simulink model "PubIfDecisionLM_MDL"  (R2020b)
settings: configuration reference "DspaceConfig" (kept outside this file)
PostLoadFcn:
  | if any(exist('dsrtsu_mdlpostloadfcn', 'file') ~= 0), dsrtsu_mdlpostloadfcn('Execute', bdroot); end
InitFcn:
  | , if any(exist('dsmpb_private', 'file') ~= 0), dsmpb_private('dsmpb_mdlclblib', 'Init', bdroot); end,
undefined symbols (not defined in the file or in its folder): OFM_OBJ_FUSIONTYPE_E, OFM_OBJ_MOVINGSTATE_E, OFM_OBJ_ORIENTATION_E, OFM_OBJ_TYPE_E, P_LM_Cyc, P_LM_EMLHistKapRcdBufSize, P_LM_EMLHistTrajBaseDis, P_LM_EMLHistTrajPNum, P_LM_EMLKapCorrMaxThre, P_LM_EMLMinKapThre, P_LM_EMLPathDisDiffThre, P_LM_EMLQuaFiltPar, P_LM_EMLTurnActKapThre, P_LM_EMLValidQuaThre, P_LM_FntPath1Disgap, P_LM_FntPath1MinDis, P_LM_FntPath1Timegap, P_LM_FntPath2Disgap, P_LM_FntPath2MinDis, P_LM_FntPath2Timegap, P_LM_FntPath3Disgap, P_LM_FntPath3MinDis, P_LM_FntPath3Timegap, P_LM_FusBLParFiltP, P_LM_FusEVDifC2Thre, P_LM_FusEVOPath1AllVSLDisThre, P_LM_FusEVOPath1AllVSLLostNumThre, P_LM_FusEVOPath1AllVSLQuaThre, P_LM_FusEVOPath1OTLFacNLC, P_LM_FusOTLQuaThre, P_LM_FusOTLSW, P_LM_FusParC0Index, P_LM_FusParC1Index, P_LM_FusParC2Index, P_LM_FusParC3Index, P_LM_FusVSLQuaThre, P_LM_FusVSLSW, P_LM_FusVSLValidSteerWheerAngThre, P_LM_FusVSLValidVxvThre, P_LM_LaneWidth, P_LM_OTLBufTPInfoEvaFactor, P_LM_OTLObjNum, P_LM_OTLObjSelectAgeThre, P_LM_OTLObjSelectDxAssessVx, P_LM_OTLObjSelectDxThre, P_LM_OTLObjSelectVxThre, P_LM_OTLObjSelectVyAssessDx, P_LM_OTLObjSelectVyThre, P_LM_OTLTrajPntBaseDis, P_LM_OTLTrajStdThre, P_LM_VSLAvailLineNum, P_LM_VSLBLSDiffThre, P_LM_VSLBLSDisRatio, P_LM_VSLFusBLParFiltP_C1, P_LM_VSLFusBLParFiltP_C2, P_LM_VSLFusBLParFiltP_C3, P_LM_VSLFusBLParFiltP_Quality, P_LM_VSLHistTrajBaseDis, P_LM_VSLHistTrajPNum, P_LM_VSLLCC0diff ... (+18)
libraries: simulink x145, LM_LIB x43
(part 4 of 24)

== system PubIfDecisionLM_MDL/Subsystem2/LM_Fusion1/LM_FusBaseLineInfoCalc/LM_FusBLRearPath ==
  LM_VSL : Inport
  Bus Creator : BusCreator  Inputs=5  OutDataTypeStr=Bus: LM_FusBLPathInfoBus
  Bus Creator1 : BusCreator  Inputs=5  OutDataTypeStr=Bus: LM_FusBLPathInfoBus
  Bus Creator2 : BusCreator  Inputs=5  OutDataTypeStr=Bus: LM_FusBLPathInfoBus
  Bus Selector : BusSelector  OutputSignals=LM_VSLRearPath1P,LM_VSLRearPath1Qulity
  Bus Selector1 : BusSelector  OutputSignals=LM_VSLRearPath2P,LM_VSLRearPath2Qulity
  Bus Selector2 : BusSelector  OutputSignals=LM_VSLRearPath3P,LM_VSLRearPath3Qulity
  LM_EMLRearPath2 : Subsystem
  LM_EMLRearPath3 : Subsystem
  LM_EMLRearPath4 : Subsystem
  Signal Conversion{1..15} (15 alike) : SignalConversion  OverrideOpt=off
  LM_FusBLRearPath1Info : Outport
  LM_FusBLRearPath2Info : Outport  Port=2
  LM_FusBLRearPath3Info : Outport  Port=3
  wires:
  Bus Selector2/2 -> LM_EMLRearPath3/2(LM_VSLRearPath3Quality)  "<LM_VSLRearPath3Qulity>"
  Bus Selector2/1 -> LM_EMLRearPath3/1(LM_VSLRearPath3P)  "<LM_VSLRearPath3P>"
  Bus Selector1/2 -> LM_EMLRearPath2/2(LM_VSLRearPath1Quality)  "<LM_VSLRearPath2Qulity>"
  Bus Selector1/1 -> LM_EMLRearPath2/1(LM_VSLRearPath2P)  "<LM_VSLRearPath2P>"
  Bus Selector/2 -> LM_EMLRearPath4/2(LM_VSLRearPath1Quality)  "<LM_VSLRearPath1Qulity>"
  Bus Selector/1 -> LM_EMLRearPath4/1(LM_VSLRearPath1P)  "<LM_VSLRearPath1P>"
  LM_VSL/1 -> Bus Selector2/1, Bus Selector1/1, Bus Selector/1
  Bus Creator2/1 -> LM_FusBLRearPath3Info/1  "LM_FusBLRearPath3Info"
  Bus Creator1/1 -> LM_FusBLRearPath2Info/1  "LM_FusBLRearPath2Info"
  Bus Creator/1 -> LM_FusBLRearPath1Info/1  "LM_FusBLRearPath1Info"
  LM_EMLRearPath4/3(LM_FusBLRearPath1C2) -> Signal Conversion11/1
  LM_EMLRearPath4/1(LM_FusBLRearPath1C0) -> Signal Conversion9/1
  LM_EMLRearPath4/2(LM_FusBLRearPath1C1) -> Signal Conversion10/1
  Signal Conversion9/1 -> Bus Creator/1  "LM_FusBLPathC0"
  Signal Conversion12/1 -> Bus Creator/4  "LM_FusBLPathC3"
  Signal Conversion10/1 -> Bus Creator/2  "LM_FusBLPathC1"
  Signal Conversion11/1 -> Bus Creator/3  "LM_FusBLPathC2"
  Signal Conversion13/1 -> Bus Creator/5  "LM_FusBLPathQuality"
  LM_EMLRearPath4/4(LM_FusBLRearPath1C3) -> Signal Conversion12/1
  LM_EMLRearPath4/5(LM_FusBLRearPath1Quality) -> Signal Conversion13/1
  LM_EMLRearPath2/5(LM_FusBLRearPath2Quality) -> Signal Conversion4/1
  LM_EMLRearPath2/4(LM_FusBLRearPath2C3) -> Signal Conversion3/1
  Signal Conversion4/1 -> Bus Creator1/5  "LM_FusBLPathQuality"
  Signal Conversion2/1 -> Bus Creator1/3  "LM_FusBLPathC2"
  Signal Conversion1/1 -> Bus Creator1/2  "LM_FusBLPathC1"
  Signal Conversion3/1 -> Bus Creator1/4  "LM_FusBLPathC3"
  Signal Conversion5/1 -> Bus Creator1/1  "LM_FusBLPathC0"
  LM_EMLRearPath2/2(LM_FusBLRearPath2C1) -> Signal Conversion1/1
  LM_EMLRearPath2/1(LM_FusBLRearPath2C0) -> Signal Conversion5/1
  LM_EMLRearPath2/3(LM_FusBLRearPath2C2) -> Signal Conversion2/1
  LM_EMLRearPath3/3(LM_FusBLRearPath3C2) -> Signal Conversion7/1
  LM_EMLRearPath3/1(LM_FusBLRearPath3C0) -> Signal Conversion15/1
  LM_EMLRearPath3/2(LM_FusBLRearPath3C1) -> Signal Conversion6/1
  Signal Conversion15/1 -> Bus Creator2/1  "LM_FusBLPathC0"
  Signal Conversion8/1 -> Bus Creator2/4  "LM_FusBLPathC3"
  Signal Conversion6/1 -> Bus Creator2/2  "LM_FusBLPathC1"
  Signal Conversion7/1 -> Bus Creator2/3  "LM_FusBLPathC2"
  Signal Conversion14/1 -> Bus Creator2/5  "LM_FusBLPathQuality"
  LM_EMLRearPath3/4(LM_FusBLRearPath3C3) -> Signal Conversion8/1
  LM_EMLRearPath3/5(LM_FusBLRearPath3Quality) -> Signal Conversion14/1

== system PubIfDecisionLM_MDL/Subsystem2/LM_Fusion1/LM_FusRatioCalc/LM_FusionCase ==
  note: 0-EML
      | 1-VSL+EML
      | 2-VSL+EML+OTL
      | 3-EML+OTL
  LM_VSLFntPaht1Quality : Inport
  LM_OTLFntPath1Qulity : Inport  Port=2
  LM_OTLFntPath2Qulity : Inport  Port=3
  LM_OTLFntPath3Qulity : Inport  Port=4
  LM_REL : Inport  Port=5
  LM_MAL : Inport  Port=6
  vxvRefMs : Inport  Port=7
  SteerWheelAng : Inport  Port=8
  LM_FusCaseJudge : Subsystem
  LM_FusCaseOTLValidJudge : Subsystem
  LM_FusCaseVSLValidJudge : Subsystem
  Terminator : Terminator
  Terminator1 : Terminator
  LM_FusCase : Outport
  wires:
  LM_REL/1 -> Terminator/1
  LM_MAL/1 -> Terminator1/1
  LM_FusCaseVSLValidJudge/1(LM_FusVSLValid) -> LM_FusCaseJudge/1(LM_FusVSLValid)
  LM_FusCaseOTLValidJudge/1(LM_FusOTLValid) -> LM_FusCaseJudge/2(LM_FusOTLValid)
  LM_FusCaseJudge/1(LM_FusCase) -> LM_FusCase/1
  SteerWheelAng/1 -> LM_FusCaseVSLValidJudge/3(SteerWheelAng)
  LM_VSLFntPaht1Quality/1 -> LM_FusCaseVSLValidJudge/1(LM_VSLFntPaht1Quality)
  vxvRefMs/1 -> LM_FusCaseVSLValidJudge/2(vxvRefMs)
  LM_OTLFntPath3Qulity/1 -> LM_FusCaseOTLValidJudge/3(LM_OTLFntPath3Qulity)
  LM_OTLFntPath2Qulity/1 -> LM_FusCaseOTLValidJudge/2(LM_OTLFntPath2Qulity)
  LM_OTLFntPath1Qulity/1 -> LM_FusCaseOTLValidJudge/1(LM_OTLFntPath1Qulity)

== system PubIfDecisionLM_MDL/Subsystem2/LM_Fusion1/LM_FusRatioCalc/LM_Fusion_EMLOnly ==
  LM_EML : Inport
  Action Port : ActionPort  ActionPortLabel=case [ 0 ]:
  Bus Creator : BusCreator  Inputs=2  OutDataTypeStr=Bus: LM_FusRatioInfoBus  NonVirtualBus=on
  Bus Creator1 : BusCreator  Inputs=4  OutDataTypeStr=Bus: LM_FusC0InfoBus  NonVirtualBus=on
  Bus Selector : BusSelector  OutputSignals=LM_EMLLLC0,LM_EMLLRC0,LM_EMLRLC0,LM_EMLRRC0
  LM_FusBaseLineC0Info : Subsystem
  LM_FusEMLAndVSLRatioCalc : Subsystem
  LM_FusBLInfo : Outport
  LM_C0Info : Outport  Port=2
  wires:
  Bus Selector/2 -> LM_FusBaseLineC0Info/2(LM_EMLC0)  "<LM_EMLLRC0>"
  Bus Selector/4 -> LM_FusBaseLineC0Info/4(LM_EMLRRC0)  "<LM_EMLRRC0>"
  Bus Selector/3 -> LM_FusBaseLineC0Info/3(LM_EMLRLC0)  "<LM_EMLRLC0>"
  LM_EML/1 -> Bus Selector/1
  Bus Creator/1 -> LM_FusBLInfo/1
  Bus Selector/1 -> LM_FusBaseLineC0Info/1(LM_EMLLLC0)  "<LM_EMLLLC0>"
  LM_FusBaseLineC0Info/1(LM_LLC0) -> Bus Creator1/1
  LM_FusBaseLineC0Info/2(LM_LRC0) -> Bus Creator1/2
  LM_FusBaseLineC0Info/3(LM_RLC0) -> Bus Creator1/3
  LM_FusBaseLineC0Info/4(LM_RRC0) -> Bus Creator1/4
  LM_FusEMLAndVSLRatioCalc/1(LM_FusFntPathK) -> Bus Creator/1
  LM_FusEMLAndVSLRatioCalc/2(LM_FusRearPathK) -> Bus Creator/2
  Bus Creator1/1 -> LM_C0Info/1  "LM_C0Info"

== system PubIfDecisionLM_MDL/Subsystem2/LM_Fusion1/LM_FusRatioCalc/LM_Fusion_EO ==
  DIR_BUS : Inport
  LM_EML : Inport  Port=2
  LM_OTL : Inport  Port=3
  LM_Com : Inport  Port=4
  LM_VIE_BUS : Inport  Port=5
  Action Port : ActionPort  ActionPortLabel=case [ 3 ]:
  Bus Creator : BusCreator  Inputs=2  OutDataTypeStr=Bus: LM_FusRatioInfoBus  NonVirtualBus=on
  Bus Creator1 : BusCreator  Inputs=4  OutDataTypeStr=Bus: LM_FusC0InfoBus  NonVirtualBus=on
  Bus Selector : BusSelector  OutputSignals=LM_EMLLLC0,LM_EMLLRC0,LM_EMLRLC0,LM_EMLRRC0
  LM_FusBaseLineC0Info : Subsystem
  LM_FusEVORatioCalc : Subsystem
  LM_FusRatioInfo : Outport
  LM_C0Info : Outport  Port=2
  wires:
  LM_VIE_BUS/1 -> LM_FusEVORatioCalc/5(LM_VIE_BUS)
  LM_OTL/1 -> LM_FusEVORatioCalc/3(LM_OTL)
  Bus Creator/1 -> LM_FusRatioInfo/1  "LM_FusRatioInfo"
  Bus Selector/4 -> LM_FusBaseLineC0Info/4(LM_VSLRRC0Adju)  "<LM_EMLRRC0>"
  LM_Com/1 -> LM_FusEVORatioCalc/4(LM_Com)
  LM_EML/1 -> Bus Selector/1, LM_FusEVORatioCalc/2(LM_EML)
  Bus Selector/2 -> LM_FusBaseLineC0Info/2(LM_VSLLRC0Adju)  "<LM_EMLLRC0>"
  Bus Selector/1 -> LM_FusBaseLineC0Info/1(LM_VSLLLC0Adju)  "<LM_EMLLLC0>"
  Bus Selector/3 -> LM_FusBaseLineC0Info/3(LM_VSLRLC0Adju)  "<LM_EMLRLC0>"
  LM_FusBaseLineC0Info/3(LM_RLC0) -> Bus Creator1/3
  Bus Creator1/1 -> LM_C0Info/1  "LM_C0Info"
  LM_FusBaseLineC0Info/4(LM_RRC0) -> Bus Creator1/4
  LM_FusBaseLineC0Info/1(LM_LLC0) -> Bus Creator1/1
  LM_FusBaseLineC0Info/2(LM_LRC0) -> Bus Creator1/2
  LM_FusEVORatioCalc/1(LM_FusFntPathK) -> Bus Creator/1
  LM_FusEVORatioCalc/2(LM_FusRearPathK) -> Bus Creator/2
  DIR_BUS/1 -> LM_FusEVORatioCalc/1(DIR_BUS)

== system PubIfDecisionLM_MDL/Subsystem2/LM_Fusion1/LM_FusRatioCalc/LM_Fusion_EV ==
  LM_VSL : Inport
  LM_EML : Inport  Port=2
  LM_VIE_BUS : Inport  Port=3
  LM_ComBus : Inport  Port=4
  DIR_BUS : Inport  Port=5
  Action Port : ActionPort  ActionPortLabel=case [ 1 ]:
  Bus Creator : BusCreator  Inputs=2  OutDataTypeStr=Bus: LM_FusRatioInfoBus  NonVirtualBus=on
  Bus Creator1 : BusCreator  Inputs=4  OutDataTypeStr=Bus: LM_FusC0InfoBus  NonVirtualBus=on
  LM_FusBaseLineC0Info : Subsystem
  LM_FusEMLAndVSLRatioCalc : Subsystem
  LM_FusBLInfo : Outport
  LM_C0Info : Outport  Port=2
  wires:
  LM_VSL/1 -> LM_FusBaseLineC0Info/2(LM_VSL), LM_FusEMLAndVSLRatioCalc/4(LM_VSL)
  LM_EML/1 -> LM_FusBaseLineC0Info/3(LM_EML), LM_FusEMLAndVSLRatioCalc/5(LM_EML)
  LM_ComBus/1 -> LM_FusEMLAndVSLRatioCalc/2(LM_ComBus)
  Bus Creator/1 -> LM_FusBLInfo/1  "LM_FusBLInfo"
  LM_FusBaseLineC0Info/4(LM_RRC0) -> Bus Creator1/4
  LM_FusBaseLineC0Info/2(LM_LRC0) -> Bus Creator1/2
  LM_FusBaseLineC0Info/3(LM_RLC0) -> Bus Creator1/3
  LM_FusBaseLineC0Info/1(LM_LLC0) -> Bus Creator1/1
  Bus Creator1/1 -> LM_C0Info/1  "LM_C0Info"
  DIR_BUS/1 -> LM_FusEMLAndVSLRatioCalc/3(DIR_BUS)
  LM_FusEMLAndVSLRatioCalc/2(LM_FusRearPathK) -> Bus Creator/2
  LM_FusEMLAndVSLRatioCalc/1(LM_FusFntPathK) -> LM_FusBaseLineC0Info/1(LM_FusFntPathK), Bus Creator/1
  LM_VIE_BUS/1 -> LM_FusEMLAndVSLRatioCalc/1(LM_VIE_BUS)

== system PubIfDecisionLM_MDL/Subsystem2/LM_Fusion1/LM_FusRatioCalc/LM_Fusion_EVO ==
  LM_VSL : Inport
  LM_EML : Inport  Port=2
  LM_OTL : Inport  Port=3
  LM_Com : Inport  Port=4
  LM_VIE_BUS : Inport  Port=5
  DIR_BUS : Inport  Port=6
  Action Port : ActionPort  ActionPortLabel=case [ 2 ]:
  Bus Creator : BusCreator  Inputs=2  OutDataTypeStr=Bus: LM_FusRatioInfoBus  NonVirtualBus=on
  Bus Creator1 : BusCreator  Inputs=4  OutDataTypeStr=Bus: LM_FusC0InfoBus  NonVirtualBus=on
  Bus Selector : BusSelector  OutputSignals=LM_VSLLLC0,LM_VSLLRC0,LM_VSLRLC0,LM_VSLRRC0
  LM_FusBaseLineC0Info : Subsystem
  LM_FusEVORatioCalc : Subsystem
  LM_FusBLInfo : Outport
  LM_C0Info : Outport  Port=2
  wires:
  Bus Selector/3 -> LM_FusBaseLineC0Info/3(LM_VSLRLC0Adju)  "<LM_VSLRLC0>"
  Bus Selector/1 -> LM_FusBaseLineC0Info/1(LM_VSLLLC0Adju)  "<LM_VSLLLC0>"
  Bus Selector/2 -> LM_FusBaseLineC0Info/2(LM_VSLLRC0Adju)  "<LM_VSLLRC0>"
  LM_EML/1 -> LM_FusEVORatioCalc/2(LM_EML)
  LM_VSL/1 -> Bus Selector/1, LM_FusEVORatioCalc/1(LM_VSL)
  LM_Com/1 -> LM_FusEVORatioCalc/4(LM_Com)
  Bus Selector/4 -> LM_FusBaseLineC0Info/4(LM_VSLRRC0Adju)  "<LM_VSLRRC0>"
  Bus Creator/1 -> LM_FusBLInfo/1  "LM_FusBLInfo"
  LM_OTL/1 -> LM_FusEVORatioCalc/3(LM_OTL)
  LM_VIE_BUS/1 -> LM_FusEVORatioCalc/5(LM_VIE_BUS)
  LM_FusEVORatioCalc/1(LM_FusFntPathK) -> Bus Creator/1
  LM_FusEVORatioCalc/2(LM_FusRearPathK) -> Bus Creator/2
  LM_FusBaseLineC0Info/3(LM_RLC0) -> Bus Creator1/3
  Bus Creator1/1 -> LM_C0Info/1  "LM_C0Info"
  LM_FusBaseLineC0Info/4(LM_RRC0) -> Bus Creator1/4
  LM_FusBaseLineC0Info/1(LM_LLC0) -> Bus Creator1/1
  LM_FusBaseLineC0Info/2(LM_LRC0) -> Bus Creator1/2
  DIR_BUS/1 -> LM_FusEVORatioCalc/6(DIR_BUS)

== system PubIfDecisionLM_MDL/Subsystem2/LM_Fusion1/LM_Fus_BLConnectivityCheck/LM_Fus_BLFntPahtConnectivityCheck ==
  LM_ComBus : Inport
  LM_FusBLInfoFilt : Inport  Port=2
  Bus Creator : BusCreator  Inputs=5  OutDataTypeStr=Bus: LM_FusBLPathInfoBus
  Bus Creator1 : BusCreator  Inputs=5  OutDataTypeStr=Bus: LM_FusBLPathInfoBus
  Bus Creator2 : BusCreator  Inputs=5  OutDataTypeStr=Bus: LM_FusBLPathInfoBus
  Bus Selector : BusSelector  OutputSignals=LM_FusBLFntPath1Info.LM_FusBLPathC0,LM_FusBLFntPath1Info.LM_FusBLPathC1,LM_FusBLFntPath1Info.LM_FusBLPathC2,LM_FusBLFntPath1Info.LM_FusBLPathC3,LM_FusBLFntPath1Info.LM_FusBLPathQuality,LM_FusBLFntPath2Info.LM_FusBLPathC0,LM_FusBLFntPath2Info.LM_FusBLPathC1,LM_FusBLFntPath2Info.LM_FusBLPathC2,LM_FusBLFntPath2Info.LM_FusBLPathC3,LM_FusBLFntPath2Info.LM_FusBLPathQuality,LM_FusBLFntPath3Info.LM_FusBLPathC0,LM_FusBLFntPath3Info.LM_FusBLPathC1,LM_FusBLFntPath3Info.LM_FusBLPathC2,LM_FusBLFntPath3Info.LM_FusBLPathC3,LM_FusBLFntPath3Info.LM_FusBLPathQuality
  Bus Selector1 : BusSelector  OutputSignals=LM_PathDisBus.LM_FntPath1Dis,LM_PathDisBus.LM_FntPath2Dis
  LM_Fus_BLFntPahtConnectivityCheck : Subsystem
  Signal Conversion{,1..14} (15 alike) : SignalConversion  OverrideOpt=off
  LM_FusBLFntPath1Info : Outport
  LM_FusBLFntPath2Info : Outport  Port=2
  LM_FusBLFntPath3Info : Outport  Port=3
  wires:
  LM_FusBLInfoFilt/1 -> Bus Selector/1
  Bus Selector/1 -> LM_Fus_BLFntPahtConnectivityCheck/1(LM_FusBLFntPath1C0)  "<LM_FusBLPathC0>"
  Bus Selector/2 -> LM_Fus_BLFntPahtConnectivityCheck/2(LM_FusBLFntPath1C1)  "<LM_FusBLPathC1>"
  Bus Selector/3 -> LM_Fus_BLFntPahtConnectivityCheck/3(LM_FusBLFntPath1C2)  "<LM_FusBLPathC2>"
  Bus Selector/4 -> LM_Fus_BLFntPahtConnectivityCheck/4(LM_FusBLFntPath1C3)  "<LM_FusBLPathC3>"
  Bus Selector/5 -> LM_Fus_BLFntPahtConnectivityCheck/5(LM_FusBLFntPath1Quality)  "<LM_FusBLPathQuality>"
  Bus Selector/6 -> LM_Fus_BLFntPahtConnectivityCheck/6(LM_FusBLFntPath2C0BefAduj)  "<LM_FusBLPathC0>"
  Bus Selector/7 -> LM_Fus_BLFntPahtConnectivityCheck/7(LM_FusBLFntPath2C1)  "<LM_FusBLPathC1>"
  Bus Selector/8 -> LM_Fus_BLFntPahtConnectivityCheck/8(LM_FusBLFntPath2C2)  "<LM_FusBLPathC2>"
  Bus Selector/9 -> LM_Fus_BLFntPahtConnectivityCheck/9(LM_FusBLFntPath2C3)  "<LM_FusBLPathC3>"
  Bus Selector/10 -> LM_Fus_BLFntPahtConnectivityCheck/10(LM_FusBLFntPath2Quality)  "<LM_FusBLPathQuality>"
  Bus Selector/11 -> LM_Fus_BLFntPahtConnectivityCheck/11(LM_FusBLFntPath3C0BefAduj)  "<LM_FusBLPathC0>"
  Bus Selector/12 -> LM_Fus_BLFntPahtConnectivityCheck/12(LM_FusBLFntPath3C1)  "<LM_FusBLPathC1>"
  Bus Selector/13 -> LM_Fus_BLFntPahtConnectivityCheck/13(LM_FusBLFntPath3C2)  "<LM_FusBLPathC2>"
  Bus Selector/14 -> LM_Fus_BLFntPahtConnectivityCheck/14(LM_FusBLFntPath3C3)  "<LM_FusBLPathC3>"
  Bus Selector/15 -> LM_Fus_BLFntPahtConnectivityCheck/15(LM_FusBLFntPath3Quality)  "<LM_FusBLPathQuality>"
  LM_ComBus/1 -> Bus Selector1/1
  Bus Selector1/1 -> LM_Fus_BLFntPahtConnectivityCheck/16(LM_FntPath1Dis)  "<LM_FntPath1Dis>"
  Bus Selector1/2 -> LM_Fus_BLFntPahtConnectivityCheck/17(LM_FntPath2Dis)  "<LM_FntPath2Dis>"
  LM_Fus_BLFntPahtConnectivityCheck/1(LM_FusBLFntPath1C0Adju) -> Signal Conversion/1
  LM_Fus_BLFntPahtConnectivityCheck/2(LM_FusBLFntPath1C1Adju) -> Signal Conversion1/1
  LM_Fus_BLFntPahtConnectivityCheck/4(LM_FusBLFntPath1C3Adju) -> Signal Conversion3/1
  LM_Fus_BLFntPahtConnectivityCheck/3(LM_FusBLFntPath1C2Adju) -> Signal Conversion2/1
  LM_Fus_BLFntPahtConnectivityCheck/7(LM_FusBLFntPath2C1Adju) -> Signal Conversion6/1
  LM_Fus_BLFntPahtConnectivityCheck/8(LM_FusBLFntPath2C2Adju) -> Signal Conversion7/1
  LM_Fus_BLFntPahtConnectivityCheck/6(LM_FusBLFntPath2C0Adju) -> Signal Conversion5/1
  LM_Fus_BLFntPahtConnectivityCheck/5(LM_FusBLFntPath1QualityAdju) -> Signal Conversion4/1
  LM_Fus_BLFntPahtConnectivityCheck/13(LM_FusBLFntPath3C2Adju) -> Signal Conversion12/1
  LM_Fus_BLFntPahtConnectivityCheck/14(LM_FusBLFntPath3C3Adju) -> Signal Conversion13/1
  LM_Fus_BLFntPahtConnectivityCheck/15(LM_FusBLFntPath3QualityAdju) -> Signal Conversion14/1
  LM_Fus_BLFntPahtConnectivityCheck/11(LM_FusBLFntPath3C0Adju) -> Signal Conversion10/1
  LM_Fus_BLFntPahtConnectivityCheck/12(LM_FusBLFntPath3C1Adju) -> Signal Conversion11/1
  LM_Fus_BLFntPahtConnectivityCheck/10(LM_FusBLFntPath2QualityAdju) -> Signal Conversion9/1
  LM_Fus_BLFntPahtConnectivityCheck/9(LM_FusBLFntPath2C3Adju) -> Signal Conversion8/1
  Bus Creator/1 -> LM_FusBLFntPath1Info/1  "LM_FusBLFntPath1Info"
  Bus Creator1/1 -> LM_FusBLFntPath2Info/1  "LM_FusBLFntPath2Info"
  Bus Creator2/1 -> LM_FusBLFntPath3Info/1  "LM_FusBLFntPath3Info"
  Signal Conversion4/1 -> Bus Creator/5  "LM_FusBLPathQuality"
  Signal Conversion3/1 -> Bus Creator/4  "LM_FusBLPathC3"
  Signal Conversion2/1 -> Bus Creator/3  "LM_FusBLPathC2"
  Signal Conversion1/1 -> Bus Creator/2  "LM_FusBLPathC1"
  Signal Conversion/1 -> Bus Creator/1  "LM_FusBLPathC0"
  Signal Conversion5/1 -> Bus Creator1/1  "LM_FusBLPathC0"
  Signal Conversion6/1 -> Bus Creator1/2  "LM_FusBLPathC1"
  Signal Conversion7/1 -> Bus Creator1/3  "LM_FusBLPathC2"
  Signal Conversion8/1 -> Bus Creator1/4  "LM_FusBLPathC3"
  Signal Conversion9/1 -> Bus Creator1/5  "LM_FusBLPathQuality"
  Signal Conversion14/1 -> Bus Creator2/5  "LM_FusBLPathQuality"
  Signal Conversion13/1 -> Bus Creator2/4  "LM_FusBLPathC3"
  Signal Conversion12/1 -> Bus Creator2/3  "LM_FusBLPathC2"
  Signal Conversion11/1 -> Bus Creator2/2  "LM_FusBLPathC1"
  Signal Conversion10/1 -> Bus Creator2/1  "LM_FusBLPathC0"

== system PubIfDecisionLM_MDL/Subsystem2/LM_Fusion1/LM_Fus_BLConnectivityCheck/LM_Fus_BLRearPahtConnectivityCheck ==
  LM_ComBus : Inport
  LM_FusBLInfoFilt : Inport  Port=2
  Bus Creator : BusCreator  Inputs=5  OutDataTypeStr=Bus: LM_FusBLPathInfoBus
  Bus Creator1 : BusCreator  Inputs=5  OutDataTypeStr=Bus: LM_FusBLPathInfoBus
  Bus Creator3 : BusCreator  Inputs=5  OutDataTypeStr=Bus: LM_FusBLPathInfoBus
  Bus Selector : BusSelector  OutputSignals=LM_FusBLRearPath1Info.LM_FusBLPathC0,LM_FusBLRearPath1Info.LM_FusBLPathC1,LM_FusBLRearPath1Info.LM_FusBLPathC2,LM_FusBLRearPath1Info.LM_FusBLPathC3,LM_FusBLRearPath1Info.LM_FusBLPathQuality,LM_FusBLRearPath2Info.LM_FusBLPathC0,LM_FusBLRearPath2Info.LM_FusBLPathC1,LM_FusBLRearPath2Info.LM_FusBLPathC2,LM_FusBLRearPath2Info.LM_FusBLPathC3,LM_FusBLRearPath2Info.LM_FusBLPathQuality,LM_FusBLRearPath3Info.LM_FusBLPathC0,LM_FusBLRearPath3Info.LM_FusBLPathC1,LM_FusBLRearPath3Info.LM_FusBLPathC2,LM_FusBLRearPath3Info.LM_FusBLPathC3,LM_FusBLRearPath3Info.LM_FusBLPathQuality
  Bus Selector1 : BusSelector  OutputSignals=LM_PathDisBus.LM_RearPath1Dis,LM_PathDisBus.LM_RearPath2Dis
  LM_Fus_BLRearPahtConnectivityCheck : Subsystem
  Signal Conversion{,1..11,14..16} (15 alike) : SignalConversion  OverrideOpt=off
  LM_FusBLFntPath1Info : Outport
  LM_FusBLFntPath2Info : Outport  Port=2
  LM_FusBLFntPath3Info : Outport  Port=3
  wires:
  LM_FusBLInfoFilt/1 -> Bus Selector/1
  Bus Selector/1 -> LM_Fus_BLRearPahtConnectivityCheck/1(LM_FusBLRearPath1C0)  "<LM_FusBLPathC0>"
  Bus Selector/2 -> LM_Fus_BLRearPahtConnectivityCheck/2(LM_FusBLRearPath1C1)  "<LM_FusBLPathC1>"
  Bus Selector/3 -> LM_Fus_BLRearPahtConnectivityCheck/3(LM_FusBLRearPath1C2)  "<LM_FusBLPathC2>"
  Bus Selector/4 -> LM_Fus_BLRearPahtConnectivityCheck/4(LM_FusBLRearPath1C3)  "<LM_FusBLPathC3>"
  Bus Selector/5 -> LM_Fus_BLRearPahtConnectivityCheck/5(LM_FusBLRearPath1Quality)  "<LM_FusBLPathQuality>"
  Bus Selector/6 -> LM_Fus_BLRearPahtConnectivityCheck/6(LM_FusBLRearPath2C0BefAduj)  "<LM_FusBLPathC0>"
  Bus Selector/7 -> LM_Fus_BLRearPahtConnectivityCheck/7(LM_FusBLRearPath2C1)  "<LM_FusBLPathC1>"
  Bus Selector/8 -> LM_Fus_BLRearPahtConnectivityCheck/8(LM_FusBLRearPath2C2)  "<LM_FusBLPathC2>"
  Bus Selector/9 -> LM_Fus_BLRearPahtConnectivityCheck/9(LM_FusBLRearPath2C3)  "<LM_FusBLPathC3>"
  Bus Selector/10 -> LM_Fus_BLRearPahtConnectivityCheck/10(LM_FusBLRearPath2Quality)  "<LM_FusBLPathQuality>"
  Bus Selector/11 -> LM_Fus_BLRearPahtConnectivityCheck/11(LM_FusBLRearPath3C0BefAduj)  "<LM_FusBLPathC0>"
  Bus Selector/12 -> LM_Fus_BLRearPahtConnectivityCheck/12(LM_FusBRearPath3C1)  "<LM_FusBLPathC1>"
  Bus Selector/13 -> LM_Fus_BLRearPahtConnectivityCheck/13(LM_FusBLRearPath3C2)  "<LM_FusBLPathC2>"
  Bus Selector/14 -> LM_Fus_BLRearPahtConnectivityCheck/14(LM_FusBLRearPath3C3)  "<LM_FusBLPathC3>"
  Bus Selector/15 -> LM_Fus_BLRearPahtConnectivityCheck/15(LM_FusBLRearPath3Quality)  "<LM_FusBLPathQuality>"
  LM_ComBus/1 -> Bus Selector1/1
  Bus Selector1/1 -> LM_Fus_BLRearPahtConnectivityCheck/16(LM_RearPath1Dis)  "<LM_RearPath1Dis>"
  Bus Selector1/2 -> LM_Fus_BLRearPahtConnectivityCheck/17(LM_RearPath2Dis)  "<LM_RearPath2Dis>"
  LM_Fus_BLRearPahtConnectivityCheck/1(LM_FusBLRearPath1C0Adju) -> Signal Conversion/1
  LM_Fus_BLRearPahtConnectivityCheck/2(LM_FusBLRearPath1C1Adju) -> Signal Conversion1/1
  LM_Fus_BLRearPahtConnectivityCheck/3(LM_FusBLRearPath1C2Adju) -> Signal Conversion2/1
  LM_Fus_BLRearPahtConnectivityCheck/6(LM_FusBLRearPath2C0Adju) -> Signal Conversion5/1
  LM_Fus_BLRearPahtConnectivityCheck/5(LM_FusBLRearPath1QualityAdju) -> Signal Conversion4/1
  LM_Fus_BLRearPahtConnectivityCheck/4(LM_FusBLRearPath1C3Adju) -> Signal Conversion3/1
  LM_Fus_BLRearPahtConnectivityCheck/10(LM_FusBLRearPath2QualityAdju) -> Signal Conversion9/1
  LM_Fus_BLRearPahtConnectivityCheck/11(LM_FusBLRearPath3C0Adju) -> Signal Conversion10/1
  LM_Fus_BLRearPahtConnectivityCheck/12(LM_FusBLRearPath3C1Adju) -> Signal Conversion11/1
  LM_Fus_BLRearPahtConnectivityCheck/9(LM_FusBLRearPath2C3Adju) -> Signal Conversion8/1
  LM_Fus_BLRearPahtConnectivityCheck/8(LM_FusBLRearPath2C2Adju) -> Signal Conversion7/1
  LM_Fus_BLRearPahtConnectivityCheck/7(LM_FusBLRearPath2C1Adju) -> Signal Conversion6/1
  LM_Fus_BLRearPahtConnectivityCheck/13(LM_FusBLRearPath3C2Adju) -> Signal Conversion14/1
  LM_Fus_BLRearPahtConnectivityCheck/14(LM_FusBLRearPath3C3Adju) -> Signal Conversion15/1
  LM_Fus_BLRearPahtConnectivityCheck/15(LM_FusBLRearPath3QualityAdju) -> Signal Conversion16/1
  Bus Creator3/1 -> LM_FusBLFntPath3Info/1  "LM_FusBLRearPath3Info"
  Bus Creator1/1 -> LM_FusBLFntPath2Info/1  "LM_FusBLRearPath2Info"
  Bus Creator/1 -> LM_FusBLFntPath1Info/1  "LM_FusBLRearPath1Info"
  Signal Conversion4/1 -> Bus Creator/5  "LM_FusBLPathQuality"
  Signal Conversion3/1 -> Bus Creator/4  "LM_FusBLPathC3"
  Signal Conversion2/1 -> Bus Creator/3  "LM_FusBLPathC2"
  Signal Conversion1/1 -> Bus Creator/2  "LM_FusBLPathC1"
  Signal Conversion/1 -> Bus Creator/1  "LM_FusBLPathC0"
  Signal Conversion5/1 -> Bus Creator1/1  "LM_FusBLPathC0"
  Signal Conversion6/1 -> Bus Creator1/2  "LM_FusBLPathC1"
  Signal Conversion7/1 -> Bus Creator1/3  "LM_FusBLPathC2"
  Signal Conversion8/1 -> Bus Creator1/4  "LM_FusBLPathC3"
  Signal Conversion9/1 -> Bus Creator1/5  "LM_FusBLPathQuality"
  Signal Conversion16/1 -> Bus Creator3/5  "LM_FusBLPathQuality"
  Signal Conversion15/1 -> Bus Creator3/4  "LM_FusBLPathC3"
  Signal Conversion14/1 -> Bus Creator3/3  "LM_FusBLPathC2"
  Signal Conversion11/1 -> Bus Creator3/2  "LM_FusBLPathC1"
  Signal Conversion10/1 -> Bus Creator3/1  "LM_FusBLPathC0"

== system PubIfDecisionLM_MDL/Subsystem2/LM_Fusion1/LM_FusfCamValidInfoCalc/LM_FusfCamValidInfoCalc ==
  LM_FusFntPath1VSLK : Inport
  LM_FusFntPath2VSLK : Inport  Port=2
  LM_FusFntPath3VSLK : Inport  Port=3
  Compare To Zero : simulink/Logic and Bit Operations/Compare To Zero  relop=~=  OutDataTypeStr=boolean
  Compare To Zero1 : simulink/Logic and Bit Operations/Compare To Zero  relop=~=  OutDataTypeStr=boolean
  Compare To Zero2 : simulink/Logic and Bit Operations/Compare To Zero  relop=~=  OutDataTypeStr=boolean
  Constant : Constant  OutDataTypeStr=uint8
  Constant1 : Constant  Value=0  OutDataTypeStr=uint8
  Switch : Switch  Criteria=u2 ~= 0
  Switch1 : Switch  Criteria=u2 ~= 0
  Switch2 : Switch  Criteria=u2 ~= 0
  LM_FusFntPath1fCamValid : Outport
  LM_FusFntPath2fCamValid : Outport  Port=2
  LM_FusFntPath3fCamValid : Outport  Port=3
  wires:
  Compare To Zero/1 -> Switch/2
  LM_FusFntPath1VSLK/1 -> Compare To Zero/1
  Compare To Zero1/1 -> Switch1/2
  Compare To Zero2/1 -> Switch2/2
  LM_FusFntPath3VSLK/1 -> Compare To Zero2/1
  LM_FusFntPath2VSLK/1 -> Compare To Zero1/1
  Constant/1 -> Switch2/1, Switch1/1, Switch/1
  Constant1/1 -> Switch/3, Switch2/3, Switch1/3
  Switch/1 -> LM_FusFntPath1fCamValid/1  "LM_FusFntPath1fCamValid"
  Switch1/1 -> LM_FusFntPath2fCamValid/1  "LM_FusFntPath2fCamValid"
  Switch2/1 -> LM_FusFntPath3fCamValid/1  "LM_FusFntPath3fCamValid"

== system PubIfDecisionLM_MDL/Subsystem2/LM_OTL/LM_OTL_MovObjTrajFit/LM_OTL_BufTPAssess ==
  LM_OTLBufTPInfoBus : Inport
  LM_OTLBufTPVectBus : Inport  Port=2
  LM_ComBus : Inport  Port=3
  LM_OTL_BufTPInfoEva : Subsystem
  LM_OTL_BufTrajEva : Subsystem
  LM_OTL_BufTrajFlg : Outport
  wires:
  LM_OTL_BufTrajEva/1(LM_OTL_BufTrajFlg) -> LM_OTL_BufTrajFlg/1
  LM_OTL_BufTPInfoEva/1(LM_OTLBufValid) -> LM_OTL_BufTrajEva/1(LM_OTLBufValid)
  LM_OTLBufTPInfoBus/1 -> LM_OTL_BufTPInfoEva/3(LM_OTLBufTPInfoBus), LM_OTL_BufTrajEva/4(ILM_OTLBufTPInfoBus)
  LM_OTLBufTPVectBus/1 -> LM_OTL_BufTPInfoEva/2(LM_OTLBufTPVectBus), LM_OTL_BufTrajEva/3(LM_OTLBufTPVectBus)
  LM_ComBus/1 -> LM_OTL_BufTPInfoEva/1(LM_ComBus), LM_OTL_BufTrajEva/2(LM_PathDisBus)

== system PubIfDecisionLM_MDL/Subsystem2/LM_OTL/LM_OTL_MovObjTrajFit/LM_OTL_TrajFit ==
  LM_OTL_BufTrajFlg : Inport
  LM_OTLBufTPVectBus : Inport  Port=2
  LM_ComBus : Inport  Port=3
  Bus Creator2 : BusCreator  Inputs=12
  Bus Selector3 : BusSelector  OutputSignals=LM_OTLBufL1SPValidPos,LM_OTLBufL2SPValidPos,LM_OTLBufE1SPValidPos,LM_OTLBufE2SPValidPos,LM_OTLBufR1SPValidPos,LM_OTLBufR2SPValidPos,LM_OTLBufL1SPLastValidPos,LM_OTLBufL2SPLastValidPos,LM_OTLBufE1SPLastValidPos,LM_OTLBufE2SPLastValidPos,LM_OTLBufR1SPLastValidPos,LM_OTLBufR2SPLastValidPos,LM_OTLBufL1TpValidNum,LM_OTLBufL2TpValidNum,LM_OTLBufE1TpValidNum,LM_OTLBufE2TpValidNum,LM_OTLBufR1TpValidNum,LM_OTLBufR2TpValidNum,LM_OTLBufL1TpLastValidNum,LM_OTLBufL2TpLastValidNum,LM_OTLBufE1TpLastValidNum,LM_OTLBufE2TpLastValidNum,LM_OTLBufR1TpLastValidNum,LM_OTLBufR2TpLastValidNum,LM_OTLBufL1Flg,LM_OTLBufL2Flg,LM_OTLBufE1Flg,LM_OTLBufE2Flg,LM_OTLBufR1Flg,LM_OTLBufR2Flg,LM_OTLBufL1LastFlg,LM_OTLBufL2LastFlg,LM_OTLBufE1LastFlg,LM_OTLBufE2LastFlg,LM_OTLBufR1LastFlg,LM_OTLBufR2LastFlg,LM_OTLBufL1Offset,LM_OTLBufL2Offset,LM_OTLBufE1Offset,LM_OTLBufE2Offset,LM_OTLBufR1Offset,LM_OTLBufR2Offset,LM_OTLBufL1LastOffset,LM_OTLBufL2LastOffset,LM_OTLBufE1LastOffset,LM_OTLBufE2LastOffset,LM_OTLBufR1LastOffset,LM_OTLBufR2LastOffset
  Bus Selector4 : BusSelector  OutputSignals=LM_OTLBufL1DxVect,LM_OTLBufL1DyVect,LM_OTLBufL2DxVect,LM_OTLBufL2DyVect,LM_OTLBufE1DxVect,LM_OTLBufE1DyVect,LM_OTLBufE2DxVect,LM_OTLBufE2DyVect,LM_OTLBufR1DxVect,LM_OTLBufR1DyVect,LM_OTLBufR2DxVect,LM_OTLBufR2DyVect
  Bus Selector5 : BusSelector  OutputSignals=LM_PathDisBus.LM_FntPath1Dis,LM_PathDisBus.LM_FntPath2Dis,LM_PathDisBus.LM_FntPath3Dis
  Constant : Constant  Value=zeros(1,4)  OutDataTypeStr=single
  Constant1 : Constant  Value=0  OutDataTypeStr=single
  Constant2 : Constant  Value=zeros(1,4)  OutDataTypeStr=single
  Constant3 : Constant  Value=0  OutDataTypeStr=single
  Constant4 : Constant  Value=zeros(1,4)  OutDataTypeStr=single
  Constant5 : Constant  Value=0  OutDataTypeStr=single
  MATLAB Function1 : MATLAB Function  TreatAsAtomicUnit=on
  MATLAB Function3 : MATLAB Function  TreatAsAtomicUnit=on
  OTLInfo : Outport
  wires:
  Bus Creator2/1 -> OTLInfo/1  "OTLInfo"
  LM_ComBus/1 -> Bus Selector5/1
  MATLAB Function1/3(LM_OTLFntPath2P) -> Bus Creator2/9  "LM_OTLFntPath2P"
  MATLAB Function1/2(LM_OTLFntPath1Qulity) -> Bus Creator2/8  "LM_OTLFntPath1Qulity"
  MATLAB Function1/1(LM_OTLFntPath1P) -> Bus Creator2/7  "LM_OTLFntPath1P"
  MATLAB Function1/5(LM_OTLFntPath3P) -> Bus Creator2/11  "LM_OTLFntPath3P"
  MATLAB Function1/6(LM_OTLFntPath3Qulity) -> Bus Creator2/12  "LM_OTLFntPath3Qulity"
  Constant/1 -> Bus Creator2/1  "LM_OTLRearPath1P"
  Constant5/1 -> Bus Creator2/6  "LM_VSLRearPath3Qulity"
  Constant1/1 -> Bus Creator2/2  "LM_VSLRearPath1Qulity"
  Constant4/1 -> Bus Creator2/5  "LM_OTLRearPath3P"
  Constant2/1 -> Bus Creator2/3  "LM_OTLRearPath2P"
  Constant3/1 -> Bus Creator2/4  "LM_VSLRearPath2Qulity"
  MATLAB Function1/4(LM_OTLFntPath2Qulity) -> Bus Creator2/10  "LM_OTLFntPath2Qulity"
  Bus Selector3/10 -> MATLAB Function3/22(LM_OTLBufE2LastSPPos)  "<LM_OTLBufE2SPLastValidPos>"
  Bus Selector3/21 -> MATLAB Function3/33(LM_OTLBufE1LastPNum)  "<LM_OTLBufE1TpLastValidNum>"
  Bus Selector3/44 -> MATLAB Function3/56(LM_OTLBufL2LastOffset)  "<LM_OTLBufL2LastOffset>"
  Bus Selector3/14 -> MATLAB Function3/26(LM_OTLBufL2PNum)  "<LM_OTLBufL2TpValidNum>"
  Bus Selector3/24 -> MATLAB Function3/36(LM_OTLBufR2LastPNum)  "<LM_OTLBufR2TpLastValidNum>"
  Bus Selector3/23 -> MATLAB Function3/35(LM_OTLBufR1LastPNum)  "<LM_OTLBufR1TpLastValidNum>"
  Bus Selector3/28 -> MATLAB Function3/40(LM_OTLBufE2Flg)  "<LM_OTLBufE2Flg>"
  Bus Selector3/19 -> MATLAB Function3/31(LM_OTLBufL1LastPNum)  "<LM_OTLBufL1TpLastValidNum>"
  Bus Selector3/18 -> MATLAB Function3/30(LM_OTLBufR2PNum)  "<LM_OTLBufR2TpValidNum>"
  Bus Selector3/13 -> MATLAB Function3/25(LM_OTLBufL1PNum)  "<LM_OTLBufL1TpValidNum>"
  Bus Selector3/12 -> MATLAB Function3/24(LM_OTLBufR2LastSPPos)  "<LM_OTLBufR2SPLastValidPos>"
  Bus Selector3/5 -> MATLAB Function3/17(LM_OTLBufR1SPPos)  "<LM_OTLBufR1SPValidPos>"
  Bus Selector4/11 -> MATLAB Function3/11(LM_OTLBufR2DxVect)  "<LM_OTLBufR2DxVect>"
  Bus Selector3/42 -> MATLAB Function3/54(LM_OTLBufR2Offset)  "<LM_OTLBufR2Offset>"
  Bus Selector3/46 -> MATLAB Function3/58(LM_OTLBufE2LastOffset)  "<LM_OTLBufE2LastOffset>"
  Bus Selector3/11 -> MATLAB Function3/23(LM_OTLBufR1LastSPPos)  "<LM_OTLBufR1SPLastValidPos>"
  Bus Selector3/40 -> MATLAB Function3/52(LM_OTLBufE2Offset)  "<LM_OTLBufE2Offset>"
  Bus Selector3/3 -> MATLAB Function3/15(LM_OTLBufE1SPPos)  "<LM_OTLBufE1SPValidPos>"
  Bus Selector3/47 -> MATLAB Function3/59(LM_OTLBufR1LastOffset)  "<LM_OTLBufR1LastOffset>"
  Bus Selector3/16 -> MATLAB Function3/28(LM_OTLBufE2PNum)  "<LM_OTLBufE2TpValidNum>"
  Bus Selector3/2 -> MATLAB Function3/14(LM_OTLBufL2SPPos)  "<LM_OTLBufL2SPValidPos>"
  Bus Selector3/29 -> MATLAB Function3/41(LM_OTLBufR1Flg)  "<LM_OTLBufR1Flg>"
  Bus Selector3/33 -> MATLAB Function3/45(LM_OTLBufE1LastFlg)  "<LM_OTLBufE1LastFlg>"
  Bus Selector3/48 -> MATLAB Function3/60(LM_OTLBufR2LastOffset)  "<LM_OTLBufR2LastOffset>"
  Bus Selector4/8 -> MATLAB Function3/8(LM_OTLBufE2DyVect)  "<LM_OTLBufE2DyVect>"
  Bus Selector3/6 -> MATLAB Function3/18(LM_OTLBufR2SPPos)  "<LM_OTLBufR2SPValidPos>"
  Bus Selector4/2 -> MATLAB Function3/2(LM_OTLBufL1DyVect)  "<LM_OTLBufL1DyVect>"
  Bus Selector3/20 -> MATLAB Function3/32(LM_OTLBufL2LastPNum)  "<LM_OTLBufL2TpLastValidNum>"
  Bus Selector3/38 -> MATLAB Function3/50(LM_OTLBufL2Offset)  "<LM_OTLBufL2Offset>"
  Bus Selector3/4 -> MATLAB Function3/16(LM_OTLBufE2SPPos)  "<LM_OTLBufE2SPValidPos>"
  Bus Selector4/6 -> MATLAB Function3/6(LM_OTLBufE1DyVect)  "<LM_OTLBufE1DyVect>"
  Bus Selector4/10 -> MATLAB Function3/10(LM_OTLBufR1DyVect)  "<LM_OTLBufR1DyVect>"
  Bus Selector3/27 -> MATLAB Function3/39(LM_OTLBufE1Flg)  "<LM_OTLBufE1Flg>"
  Bus Selector3/45 -> MATLAB Function3/57(LM_OTLBufE1LastOffset)  "<LM_OTLBufE1LastOffset>"
  Bus Selector4/4 -> MATLAB Function3/4(LM_OTLBufL2DyVect)  "<LM_OTLBufL2DyVect>"
  Bus Selector3/32 -> MATLAB Function3/44(LM_OTLBufL2LastFlg)  "<LM_OTLBufL2LastFlg>"
  Bus Selector3/9 -> MATLAB Function3/21(LM_OTLBufE1LastSPPos)  "<LM_OTLBufE1SPLastValidPos>"
  Bus Selector3/8 -> MATLAB Function3/20(LM_OTLBufL2LastSPPos)  "<LM_OTLBufL2SPLastValidPos>"
  Bus Selector3/25 -> MATLAB Function3/37(LM_OTLBufL1Flg)  "<LM_OTLBufL1Flg>"
  Bus Selector4/12 -> MATLAB Function3/12(LM_OTLBufR2DyVect)  "<LM_OTLBufR2DyVect>"
  Bus Selector3/37 -> MATLAB Function3/49(LM_OTLBufL1Offset)  "<LM_OTLBufL1Offset>"
  Bus Selector3/1 -> MATLAB Function3/13(LM_OTLBufL1SPPos)  "<LM_OTLBufL1SPValidPos>"
  Bus Selector3/36 -> MATLAB Function3/48(LM_OTLBufR2LastFlg)  "<LM_OTLBufR2LastFlg>"
  Bus Selector3/22 -> MATLAB Function3/34(LM_OTLBufE2LastPNum)  "<LM_OTLBufE2TpLastValidNum>"
  Bus Selector3/17 -> MATLAB Function3/29(LM_OTLBufR1PNum)  "<LM_OTLBufR1TpValidNum>"
  Bus Selector3/31 -> MATLAB Function3/43(LM_OTLBufL1LastFlg)  "<LM_OTLBufL1LastFlg>"
  Bus Selector4/9 -> MATLAB Function3/9(LM_OTLBufR1DxVect)  "<LM_OTLBufR1DxVect>"
  Bus Selector3/35 -> MATLAB Function3/47(LM_OTLBufR1LastFlg)  "<LM_OTLBufR1LastFlg>"
  Bus Selector3/15 -> MATLAB Function3/27(LM_OTLBufE1PNum)  "<LM_OTLBufE1TpValidNum>"
  Bus Selector3/34 -> MATLAB Function3/46(LM_OTLBufE2LastFlg)  "<LM_OTLBufE2LastFlg>"
  Bus Selector3/30 -> MATLAB Function3/42(LM_OTLBufR2Flg)  "<LM_OTLBufR2Flg>"
  Bus Selector4/7 -> MATLAB Function3/7(LM_OTLBufE2DxVect)  "<LM_OTLBufE2DxVect>"
  Bus Selector3/7 -> MATLAB Function3/19(LM_OTLBufL1LastSPPos)  "<LM_OTLBufL1SPLastValidPos>"
  Bus Selector3/43 -> MATLAB Function3/55(LM_OTLBufL1LastOffset)  "<LM_OTLBufL1LastOffset>"
  Bus Selector4/1 -> MATLAB Function3/1(LM_OTLBufL1DxVect)  "<LM_OTLBufL1DxVect>"
  Bus Selector4/3 -> MATLAB Function3/3(LM_OTLBufL2DxVect)  "<LM_OTLBufL2DxVect>"
  Bus Selector4/5 -> MATLAB Function3/5(LM_OTLBufE1DxVect)  "<LM_OTLBufE1DxVect>"
  Bus Selector3/26 -> MATLAB Function3/38(LM_OTLBufL2Flg)  "<LM_OTLBufL2Flg>"
  LM_OTLBufTPVectBus/1 -> Bus Selector4/1
  LM_OTL_BufTrajFlg/1 -> Bus Selector3/1
  Bus Selector3/39 -> MATLAB Function3/51(LM_OTLBufE1Offset)  "<LM_OTLBufE1Offset>"
  Bus Selector3/41 -> MATLAB Function3/53(LM_OTLBufR1Offset)  "<LM_OTLBufR1Offset>"
  Bus Selector5/1 -> MATLAB Function1/3(LM_FntPath1Dis)  "<LM_FntPath1Dis>"
  Bus Selector5/2 -> MATLAB Function1/4(LM_FntPath2Dis)  "<LM_FntPath2Dis>"
  Bus Selector5/3 -> MATLAB Function1/5(LM_FntPath3Dis)  "<LM_FntPath3Dis>"
  MATLAB Function3/1(LM_OTLBufResampeFntPathDxInfo) -> MATLAB Function1/1(LM_OTLBufResampeFntPathDxInfo)
  MATLAB Function3/2(LM_OTLBufResampeFntPathDyInfo) -> MATLAB Function1/2(LM_OTLBufResampeFntPathDyInfo)

== system PubIfDecisionLM_MDL/Subsystem2/LM_OTL/LM_OTL_MovObjTrajRecord3/LM_OTL_BufLostObjTPValidJudge ==
  LM_OTLRcdObjLostFlg_Bus : Inport
  LM_OTLBufTPInfoBusK1 : Inport  Port=2
  LM_OTLBufTPVectAdjuBus : Inport  Port=3
  Bus Creator{,1..5} (6 alike) : BusCreator  Inputs=4
  Bus Creator6 : BusCreator  Inputs=6
  Bus Selector : BusSelector  OutputSignals=LM_OTLBufLastTPValid.LM_OTLBufL1LastTPValid,LM_OTLBufLastPNumInfo.LM_OTLBufL1LastPNum,LM_OTLBufLastSPPosInfo.LM_OTLBufL1LastSPPos,LM_OTLBufLastEPPosInfo.LM_OTLBufL1LastEPPos,LM_OTLBufPNumInfo.LM_OTLBufL1PNum,LM_OTLBufSPPosInfo.LM_OTLBufL1SPPos,LM_OTLBufEPPosInfo.LM_OTLBufL1EPPos
  Bus Selector1 : BusSelector  OutputSignals=LM_OTLBufLe1ObjLostFlg
  Bus Selector10 : BusSelector  OutputSignals=LM_OTLBufRig2ObjLostFlg
  Bus Selector11 : BusSelector  OutputSignals=LM_OTLBufLastTPValid.LM_OTLBufR2LastTPValid,LM_OTLBufLastPNumInfo.LM_OTLBufR2LastPNum,LM_OTLBufLastSPPosInfo.LM_OTLBufR2LastSPPos,LM_OTLBufLastEPPosInfo.LM_OTLBufR2LastEPPos,LM_OTLBufPNumInfo.LM_OTLBufR2PNum,LM_OTLBufSPPosInfo.LM_OTLBufR2SPPos,LM_OTLBufEPPosInfo.LM_OTLBufR2EPPos
  Bus Selector12 : BusSelector  OutputSignals=LM_OTLBufL1DxVectK1Adju
  Bus Selector13 : BusSelector  OutputSignals=LM_OTLBufL2DxVectK1Adju
  Bus Selector14 : BusSelector  OutputSignals=LM_OTLBufE1DxVectK1Adju
  Bus Selector15 : BusSelector  OutputSignals=LM_OTLBufE2DxVectK1Adju
  Bus Selector16 : BusSelector  OutputSignals=LM_OTLBufR1DxVectK1Adju
  Bus Selector17 : BusSelector  OutputSignals=LM_OTLBufR2DxVectK1Adju
  Bus Selector2 : BusSelector  OutputSignals=LM_OTLBufLe2ObjLostFlg
  Bus Selector3 : BusSelector  OutputSignals=LM_OTLBufLastTPValid.LM_OTLBufL2LastTPValid,LM_OTLBufLastPNumInfo.LM_OTLBufL2LastPNum,LM_OTLBufLastSPPosInfo.LM_OTLBufL2LastSPPos,LM_OTLBufLastEPPosInfo.LM_OTLBufL2LastEPPos,LM_OTLBufPNumInfo.LM_OTLBufL2PNum,LM_OTLBufSPPosInfo.LM_OTLBufL2SPPos,LM_OTLBufEPPosInfo.LM_OTLBufL2EPPos
  Bus Selector4 : BusSelector  OutputSignals=LM_OTLBufEgo1ObjLostFlg
  Bus Selector5 : BusSelector  OutputSignals=LM_OTLBufLastTPValid.LM_OTLBufE1LastTPValid,LM_OTLBufLastPNumInfo.LM_OTLBufE1LastPNum,LM_OTLBufLastSPPosInfo.LM_OTLBufE1LastSPPos,LM_OTLBufLastEPPosInfo.LM_OTLBufE1LastEPPos,LM_OTLBufPNumInfo.LM_OTLBufE1PNum,LM_OTLBufSPPosInfo.LM_OTLBufE1SPPos,LM_OTLBufEPPosInfo.LM_OTLBufE1EPPos
  Bus Selector6 : BusSelector  OutputSignals=LM_OTLBufEgo1ObjLostFlg
  Bus Selector7 : BusSelector  OutputSignals=LM_OTLBufLastTPValid.LM_OTLBufE2LastTPValid,LM_OTLBufLastPNumInfo.LM_OTLBufE2LastPNum,LM_OTLBufLastSPPosInfo.LM_OTLBufE2LastSPPos,LM_OTLBufLastEPPosInfo.LM_OTLBufE2LastEPPos,LM_OTLBufPNumInfo.LM_OTLBufE2PNum,LM_OTLBufSPPosInfo.LM_OTLBufE2SPPos,LM_OTLBufEPPosInfo.LM_OTLBufE2EPPos
  Bus Selector8 : BusSelector  OutputSignals=LM_OTLBufRig1ObjLostFlg
  Bus Selector9 : BusSelector  OutputSignals=LM_OTLBufLastTPValid.LM_OTLBufR1LastTPValid,LM_OTLBufLastPNumInfo.LM_OTLBufR1LastPNum,LM_OTLBufLastSPPosInfo.LM_OTLBufR1LastSPPos,LM_OTLBufLastEPPosInfo.LM_OTLBufR1LastEPPos,LM_OTLBufPNumInfo.LM_OTLBufR1PNum,LM_OTLBufSPPosInfo.LM_OTLBufR1SPPos,LM_OTLBufEPPosInfo.LM_OTLBufR1EPPos
  LM_OTLBufEgo1LostTPValidJudge : LM_LIB/LM_OTLBufLostTPValidJudgeNew  SystemSampleTime=-1  VariantActivationTime=update diagram  Latency=0  AutoFrameSizeCalculation=off
  LM_OTLBufEgo2LostTPValidJudge : LM_LIB/LM_OTLBufLostTPValidJudgeNew  SystemSampleTime=-1  VariantActivationTime=update diagram  Latency=0  AutoFrameSizeCalculation=off
  LM_OTLBufLe1LostTPValidJudge : LM_LIB/LM_OTLBufLostTPValidJudgeNew  SystemSampleTime=-1  VariantActivationTime=update diagram  Latency=0  AutoFrameSizeCalculation=off
  LM_OTLBufLe2LostTPValidJudge : LM_LIB/LM_OTLBufLostTPValidJudgeNew  SystemSampleTime=-1  VariantActivationTime=update diagram  Latency=0  AutoFrameSizeCalculation=off
  LM_OTLBufRig1LostTPValidJudge : LM_LIB/LM_OTLBufLostTPValidJudgeNew  SystemSampleTime=-1  VariantActivationTime=update diagram  Latency=0  AutoFrameSizeCalculation=off
  LM_OTLBufRig2LostTPValidJudge : LM_LIB/LM_OTLBufLostTPValidJudgeNew  SystemSampleTime=-1  VariantActivationTime=update diagram  Latency=0  AutoFrameSizeCalculation=off
  Signal Conversion{,1..23} (24 alike) : SignalConversion  OverrideOpt=off
  LM_OTLBufLastTPInfoBus : Outport
  wires:
  Bus Selector17/1 -> LM_OTLBufRig2LostTPValidJudge/1  "<LM_OTLBufR2DxVectK1Adju>"
  Bus Selector16/1 -> LM_OTLBufRig1LostTPValidJudge/1  "<LM_OTLBufR1DxVectK1Adju>"
  Bus Selector15/1 -> LM_OTLBufEgo2LostTPValidJudge/1  "<LM_OTLBufE2DxVectK1Adju>"
  Bus Selector14/1 -> LM_OTLBufEgo1LostTPValidJudge/1  "<LM_OTLBufE1DxVectK1Adju>"
  Bus Selector13/1 -> LM_OTLBufLe2LostTPValidJudge/1  "<LM_OTLBufL2DxVectK1Adju>"
  Bus Selector12/1 -> LM_OTLBufLe1LostTPValidJudge/1  "<LM_OTLBufL1DxVectK1Adju>"
  LM_OTLBufTPVectAdjuBus/1 -> Bus Selector12/1, Bus Selector13/1, Bus Selector14/1, Bus Selector15/1, Bus Selector16/1, Bus Selector17/1
  Bus Selector1/1 -> LM_OTLBufLe1LostTPValidJudge/2  "<LM_OTLBufLe1ObjLostFlg>"
  Bus Selector/1 -> LM_OTLBufLe1LostTPValidJudge/3  "<LM_OTLBufL1LastTPValid>"
  Bus Selector/2 -> LM_OTLBufLe1LostTPValidJudge/4  "<LM_OTLBufL1LastPNum>"
  Bus Selector/3 -> LM_OTLBufLe1LostTPValidJudge/5  "<LM_OTLBufL1LastSPPos>"
  Bus Selector/4 -> LM_OTLBufLe1LostTPValidJudge/6  "<LM_OTLBufL1LastEPPos>"
  Bus Selector/5 -> LM_OTLBufLe1LostTPValidJudge/7  "<LM_OTLBufL1PNum>"
  Bus Selector/6 -> LM_OTLBufLe1LostTPValidJudge/8  "<LM_OTLBufL1SPPos>"
  Bus Selector/7 -> LM_OTLBufLe1LostTPValidJudge/9  "<LM_OTLBufL1EPPos>"
  Bus Selector2/1 -> LM_OTLBufLe2LostTPValidJudge/2  "<LM_OTLBufLe2ObjLostFlg>"
  Bus Selector3/1 -> LM_OTLBufLe2LostTPValidJudge/3  "<LM_OTLBufL2LastTPValid>"
  Bus Selector3/2 -> LM_OTLBufLe2LostTPValidJudge/4  "<LM_OTLBufL2LastPNum>"
  Bus Selector3/3 -> LM_OTLBufLe2LostTPValidJudge/5  "<LM_OTLBufL2LastSPPos>"
  Bus Selector3/4 -> LM_OTLBufLe2LostTPValidJudge/6  "<LM_OTLBufL2LastEPPos>"
  Bus Selector3/5 -> LM_OTLBufLe2LostTPValidJudge/7  "<LM_OTLBufL2PNum>"
  Bus Selector3/6 -> LM_OTLBufLe2LostTPValidJudge/8  "<LM_OTLBufL2SPPos>"
  Bus Selector3/7 -> LM_OTLBufLe2LostTPValidJudge/9  "<LM_OTLBufL2EPPos>"
  Bus Selector5/7 -> LM_OTLBufEgo1LostTPValidJudge/9  "<LM_OTLBufE1EPPos>"
  Bus Selector5/6 -> LM_OTLBufEgo1LostTPValidJudge/8  "<LM_OTLBufE1SPPos>"
  Bus Selector5/5 -> LM_OTLBufEgo1LostTPValidJudge/7  "<LM_OTLBufE1PNum>"
  Bus Selector5/4 -> LM_OTLBufEgo1LostTPValidJudge/6  "<LM_OTLBufE1LastEPPos>"
  Bus Selector5/3 -> LM_OTLBufEgo1LostTPValidJudge/5  "<LM_OTLBufE1LastSPPos>"
  Bus Selector5/2 -> LM_OTLBufEgo1LostTPValidJudge/4  "<LM_OTLBufE1LastPNum>"
  Bus Selector5/1 -> LM_OTLBufEgo1LostTPValidJudge/3  "<LM_OTLBufE1LastTPValid>"
  Bus Selector4/1 -> LM_OTLBufEgo1LostTPValidJudge/2  "<LM_OTLBufEgo1ObjLostFlg>"
  LM_OTLBufLe1LostTPValidJudge/1 -> Signal Conversion/1
  LM_OTLBufLe1LostTPValidJudge/2 -> Signal Conversion1/1
  LM_OTLBufLe1LostTPValidJudge/3 -> Signal Conversion2/1
  LM_OTLBufLe1LostTPValidJudge/4 -> Signal Conversion3/1
  LM_OTLBufLe2LostTPValidJudge/4 -> Signal Conversion7/1
  LM_OTLBufLe2LostTPValidJudge/3 -> Signal Conversion6/1
  LM_OTLBufLe2LostTPValidJudge/2 -> Signal Conversion5/1
  LM_OTLBufLe2LostTPValidJudge/1 -> Signal Conversion4/1
  LM_OTLBufEgo1LostTPValidJudge/1 -> Signal Conversion8/1
  LM_OTLBufEgo1LostTPValidJudge/2 -> Signal Conversion9/1
  LM_OTLBufEgo1LostTPValidJudge/3 -> Signal Conversion10/1
  LM_OTLBufEgo1LostTPValidJudge/4 -> Signal Conversion11/1
  Bus Selector6/1 -> LM_OTLBufEgo2LostTPValidJudge/2  "<LM_OTLBufEgo1ObjLostFlg>"
  Bus Selector7/1 -> LM_OTLBufEgo2LostTPValidJudge/3  "<LM_OTLBufE2LastTPValid>"
  Bus Selector7/2 -> LM_OTLBufEgo2LostTPValidJudge/4  "<LM_OTLBufE2LastPNum>"
  Bus Selector7/3 -> LM_OTLBufEgo2LostTPValidJudge/5  "<LM_OTLBufE2LastSPPos>"
  Bus Selector7/4 -> LM_OTLBufEgo2LostTPValidJudge/6  "<LM_OTLBufE2LastEPPos>"
  Bus Selector7/5 -> LM_OTLBufEgo2LostTPValidJudge/7  "<LM_OTLBufE2PNum>"
  Bus Selector7/6 -> LM_OTLBufEgo2LostTPValidJudge/8  "<LM_OTLBufE2SPPos>"
  Bus Selector7/7 -> LM_OTLBufEgo2LostTPValidJudge/9  "<LM_OTLBufE2EPPos>"
  Bus Selector9/7 -> LM_OTLBufRig1LostTPValidJudge/9  "<LM_OTLBufR1EPPos>"
  Bus Selector9/6 -> LM_OTLBufRig1LostTPValidJudge/8  "<LM_OTLBufR1SPPos>"
  Bus Selector9/5 -> LM_OTLBufRig1LostTPValidJudge/7  "<LM_OTLBufR1PNum>"
  Bus Selector9/4 -> LM_OTLBufRig1LostTPValidJudge/6  "<LM_OTLBufR1LastEPPos>"
  Bus Selector9/3 -> LM_OTLBufRig1LostTPValidJudge/5  "<LM_OTLBufR1LastSPPos>"
  Bus Selector9/2 -> LM_OTLBufRig1LostTPValidJudge/4  "<LM_OTLBufR1LastPNum>"
  Bus Selector9/1 -> LM_OTLBufRig1LostTPValidJudge/3  "<LM_OTLBufR1LastTPValid>"
  Bus Selector8/1 -> LM_OTLBufRig1LostTPValidJudge/2  "<LM_OTLBufRig1ObjLostFlg>"
  LM_OTLBufTPInfoBusK1/1 -> Bus Selector3/1, Bus Selector5/1, Bus Selector7/1, Bus Selector9/1, Bus Selector11/1, Bus Selector/1
  LM_OTLRcdObjLostFlg_Bus/1 -> Bus Selector2/1, Bus Selector4/1, Bus Selector8/1, Bus Selector10/1, Bus Selector6/1, Bus Selector1/1
  Bus Selector10/1 -> LM_OTLBufRig2LostTPValidJudge/2  "<LM_OTLBufRig2ObjLostFlg>"
  Bus Selector11/1 -> LM_OTLBufRig2LostTPValidJudge/3  "<LM_OTLBufR2LastTPValid>"
  Bus Selector11/2 -> LM_OTLBufRig2LostTPValidJudge/4  "<LM_OTLBufR2LastPNum>"
  Bus Selector11/3 -> LM_OTLBufRig2LostTPValidJudge/5  "<LM_OTLBufR2LastSPPos>"
  Bus Selector11/4 -> LM_OTLBufRig2LostTPValidJudge/6  "<LM_OTLBufR2LastEPPos>"
  Bus Selector11/5 -> LM_OTLBufRig2LostTPValidJudge/7  "<LM_OTLBufR2PNum>"
  Bus Selector11/6 -> LM_OTLBufRig2LostTPValidJudge/8  "<LM_OTLBufR2SPPos>"
  Bus Selector11/7 -> LM_OTLBufRig2LostTPValidJudge/9  "<LM_OTLBufR2EPPos>"
  Signal Conversion1/1 -> Bus Creator/2  "LM_OTLBufL1LastPNum"
  Signal Conversion/1 -> Bus Creator/1  "LM_OTLBufL1LastTPValid"
  Signal Conversion2/1 -> Bus Creator/3  "LM_OTLBufL1LastSPPos"
  Signal Conversion3/1 -> Bus Creator/4  "LM_OTLBufL1LastEPPos"
  Signal Conversion7/1 -> Bus Creator1/4  "LM_OTLBufL2LastEPPos"
  Signal Conversion6/1 -> Bus Creator1/3  "LM_OTLBufL2LastSPPos"
  Signal Conversion4/1 -> Bus Creator1/1  "LM_OTLBufL2LastTPValid"
  Signal Conversion5/1 -> Bus Creator1/2  "LM_OTLBufL2LastPNum"
  Signal Conversion9/1 -> Bus Creator2/2  "LM_OTLBufE1LastPNum"
  Signal Conversion8/1 -> Bus Creator2/1  "LM_OTLBufE1LastTPValid"
  Signal Conversion10/1 -> Bus Creator2/3  "LM_OTLBufE1LastSPPos"
  Signal Conversion11/1 -> Bus Creator2/4  "LM_OTLBufE1LastEPPos"
  Signal Conversion15/1 -> Bus Creator5/4  "LM_OTLBufR2LastEPPos"
  Signal Conversion14/1 -> Bus Creator5/3  "LM_OTLBufR2LastSPPos"
  Signal Conversion22/1 -> Bus Creator5/1  "LM_OTLBufR2LastTPValid"
  Signal Conversion23/1 -> Bus Creator5/2  "LM_OTLBufR2LastPNum"
  Signal Conversion19/1 -> Bus Creator4/2  "LM_OTLBufR1LastPNum"
  Signal Conversion18/1 -> Bus Creator4/1  "LM_OTLBufR1LastTPValid"
  Signal Conversion20/1 -> Bus Creator4/3  "LM_OTLBufR1LastSPPos"
  Signal Conversion21/1 -> Bus Creator4/4  "LM_OTLBufR1LastEPPos"
  Signal Conversion17/1 -> Bus Creator3/4  "LM_OTLBufE2LastEPPos"
  Signal Conversion16/1 -> Bus Creator3/3  "LM_OTLBufE2LastSPPos"
  Signal Conversion12/1 -> Bus Creator3/1  "LM_OTLBufE2LastTPValid"
  Signal Conversion13/1 -> Bus Creator3/2  "LM_OTLBufE2LastPNum"
  LM_OTLBufRig2LostTPValidJudge/4 -> Signal Conversion15/1
  LM_OTLBufRig2LostTPValidJudge/3 -> Signal Conversion14/1
  LM_OTLBufRig2LostTPValidJudge/2 -> Signal Conversion23/1
  LM_OTLBufRig2LostTPValidJudge/1 -> Signal Conversion22/1
  LM_OTLBufRig1LostTPValidJudge/1 -> Signal Conversion18/1
  LM_OTLBufRig1LostTPValidJudge/2 -> Signal Conversion19/1
  LM_OTLBufRig1LostTPValidJudge/3 -> Signal Conversion20/1
  LM_OTLBufRig1LostTPValidJudge/4 -> Signal Conversion21/1
  LM_OTLBufEgo2LostTPValidJudge/4 -> Signal Conversion17/1
  LM_OTLBufEgo2LostTPValidJudge/3 -> Signal Conversion16/1
  LM_OTLBufEgo2LostTPValidJudge/2 -> Signal Conversion13/1
  LM_OTLBufEgo2LostTPValidJudge/1 -> Signal Conversion12/1
  Bus Creator5/1 -> Bus Creator6/6  "LM_OTLBufR2LastTPInfo"
  Bus Creator4/1 -> Bus Creator6/5  "LM_OTLBufR1LastTPInfo"
  Bus Creator/1 -> Bus Creator6/1  "LM_OTLBufL1LastTPInfo"
  Bus Creator1/1 -> Bus Creator6/2  "LM_OTLBufL2LastTPInfo"
  Bus Creator2/1 -> Bus Creator6/3  "LM_OTLBufE1LastTPInfo"
  Bus Creator3/1 -> Bus Creator6/4  "LM_OTLBufE2LastTPInfo"
  Bus Creator6/1 -> LM_OTLBufLastTPInfoBus/1  "LM_OTLBufLastTPInfoBus"

== system PubIfDecisionLM_MDL/Subsystem2/LM_OTL/LM_OTL_MovObjTrajRecord3/LM_OTL_BufRcdObjLostJudge ==
  note: 判断当前周期感兴趣目标是否已经存储
  LM_OTLInterestObjIndexVect : Inport
  LM_OTLRcdObjIDVectK1 : Inport  Port=2
  Object_ID : Inport  Port=3  BusOutputAsStruct=on
  Bus Creator : BusCreator  Inputs=6
  LM_OTL_EgoLaRcdObjLostJudge : Subsystem
  LM_OTL_LeLaRcdObjLostJudge : Subsystem
  LM_OTL_RigLaRcdObjLostJudge : Subsystem
  LM_OTLRcdObjLostFlg_Bus : Outport
  wires:
  LM_OTL_EgoLaRcdObjLostJudge/2(LM_OTLBufEgo2ObjLostFlg) -> Bus Creator/4
  LM_OTL_EgoLaRcdObjLostJudge/1(LM_OTLBufEgo1ObjLostFlg) -> Bus Creator/3
  LM_OTL_LeLaRcdObjLostJudge/1(LM_OTLBufLe1ObjLostFlg) -> Bus Creator/1
  LM_OTLRcdObjIDVectK1/1 -> LM_OTL_LeLaRcdObjLostJudge/2(LM_OTLRcdObjIDVectK1), LM_OTL_EgoLaRcdObjLostJudge/2(LM_OTLRcdObjIDVectK1), LM_OTL_RigLaRcdObjLostJudge/2(LM_OTLRcdObjIDVectK1)
  LM_OTL_RigLaRcdObjLostJudge/1(LM_OTLBufRig1ObjLostFlg) -> Bus Creator/5
  LM_OTL_LeLaRcdObjLostJudge/2(LM_OTLBufLe2ObjLostFlg) -> Bus Creator/2
  Bus Creator/1 -> LM_OTLRcdObjLostFlg_Bus/1  "LM_OTLRcdObjLostFlg_Bus"
  Object_ID/1 -> LM_OTL_LeLaRcdObjLostJudge/1(Object_ID), LM_OTL_EgoLaRcdObjLostJudge/1(Object_ID), LM_OTL_RigLaRcdObjLostJudge/1(Object_ID)
  LM_OTLInterestObjIndexVect/1 -> LM_OTL_LeLaRcdObjLostJudge/3(LM_OTLInterestObjIndexVect), LM_OTL_EgoLaRcdObjLostJudge/3(LM_OTLInterestObjIndexVect), LM_OTL_RigLaRcdObjLostJudge/3(LM_OTLInterestObjIndexVect)
  LM_OTL_RigLaRcdObjLostJudge/2(LM_OTLBufRig2ObjLostFlg) -> Bus Creator/6
